simulink model "Lab3_PlantModel"  (R2020a)
settings: Solver=VariableStepAuto  StartTime=0.0  StopTime=2  RelTol=1e-3
libraries: fl_lib x12, ee_lib x10, nesl_utility x3, sdl_lib x2
settings Model: Creator=stevi  LastModifiedBy=Minkyun

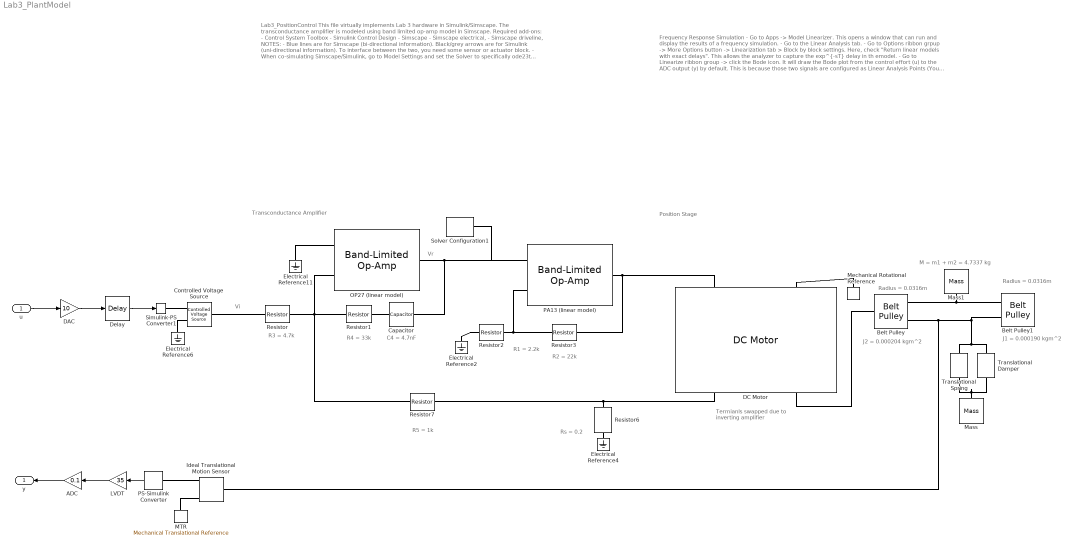
== system Lab3_PlantModel ==
  note: Position Stage
  note: Frequency Response Simulation
      |
      | - Go to Apps -> Model Linearizer. This opens a window that can run and display the results of a frequency simulation.
      | - Go to the Linear Analysis tab.
      | - Go to Options ribbon grpup -> More Options button -> Linearization tab > Block by block settings. Here, check "Return linear models with exact delays". This allows the analyzer to capture the exp^{-sT} delay in th emodel.
      | - Go to Linearize ribbon group -> click the Bode icon.
      |
      | It will draw the Bode plot from the control effort (u) to the ADC output (y) by default. This is because those two signals are configured as Linear Analysis Points (You can see little icons on top of those signal lines). To select input and output locations on block diagram...
      | - Right click on a black/grey simulink signal line. Go to Linear Analysis Points -> Select appropriate types (e.g., open-loop input or open-loop output )
      | - Select different positions for the input and output depending on which frequency response you are interested in.
      | - You just need to select input and output points on the model once and select the analysis you are interested in (e.g., Bode plot, step response, impulse response, nyquist plot, pole-zero plot etc).
      | - Run your analysis, and view the results in this window. By right clicking on the graph, you can add a background grid, change axis limits, change units, and set the phase offset (sometimes the phase will be starting from 360° rather than 0°.
  note: Lab3_PositionControl
      |
      | This file virtually implements Lab 3 hardware in Simulink/Simscape. The transconductance amplifier is modeled using band limited op-amp model in Simscape.
      |
      | Required add-ons:
      | - Control System Toolbox
      | - Simulink Control Design
      | - Simscape
      | - Simscape electrical,
      | - Simscape driveline,
      |
      | NOTES:
      | - Blue lines are for Simscape (bi-directional information). Black/grey arrows are for Simulink (uni-directional information). To interface between the two, you need some sensor or actuator block.
      | - When co-simulating Simscape/Simulink, go to Model Settings and set the Solver to specifically ode23t (mod. stiff/Trapezoidal)
      | - Following recommendation made here: https://www.mathworks.com/help/physmod/simscape/ug/creating-and-simulating-a-simple-model.html
      | - The model simulated fine under the default auto solver selection for an open-loop model, but simulated very slowly for a closed loop model.
  note: Termianls swapped due
      |  to inverting amplifier
  note: Radius = 0.0316m
  note: Vi
  note: J2 = 0.000204 kgm^2
  note: M = m1 + m2 = 4.7337 kg
  note: J1 = 0.000190 kgm^2
  note: Radius = 0.0316m
  note: R5 = 1k
  note: Vr
  note: R4 = 33k
  note: C4 = 4.7nF
  note: R1 = 2.2k
  note: Rs = 0.2
  note: Transconductance Amplifier
  note: R3 = 4.7k
  note: R2 = 22k
  u : Inport
  ADC : Gain  Gain=0.1
  Belt Pulley : sdl_lib/Couplings & Drives/Belt Pulley  belt_type=sdl.enum.belt_type.ideal  sheave_ang=30 deg  num_belts=1  model_f_c=sdl.enum.model_centrifugal.off  linear_density=0.6 kg/m  belt_direction=sdl.enum.belt_direction.opposite  breakable=sdl.enum.max_tension.off  F_max=1e5 N  check_tension=sdl.enum.tension_check.off  r_pulley=0.0316 m  b_pulley=0.01 N*m/(rad/s)  model_inertia=sdl.enum.model_inertia.on  pulley_inertia=0.000204 kg*m^2  initial_velocity=0 rad/s  mu=0.5  phi_wrap=180 deg  v_thr=0.001 m/s
      settings: SourceProductBaseCode=LD  InternalSimscapePortConfiguration="{\"Bottom\":[],\"Left\":[{\"id\":\"S\",\"label\":\"S\",\"type\":\"foundation.mechanical.rotational.rotational\"}],\"Right\":[{\"id\":\"A\",\"label\":\"A\",\"type\":\"foundation.mechanical.translational.translational\"},{\"id\":\"B\",\"label\":\"B\",\"type\":\"foundation.mechanical.translational.translational\"}],\"Top\":[]}"
  Belt Pulley1 : sdl_lib/Couplings & Drives/Belt Pulley  belt_type=sdl.enum.belt_type.ideal  sheave_ang=30 deg  num_belts=1  model_f_c=sdl.enum.model_centrifugal.off  linear_density=0.6 kg/m  belt_direction=sdl.enum.belt_direction.opposite  breakable=sdl.enum.max_tension.off  F_max=1e5 N  check_tension=sdl.enum.tension_check.off  r_pulley=0.0316 m  b_pulley=0.01 N*m/(rad/s)  model_inertia=sdl.enum.model_inertia.on  pulley_inertia=0.000190 kg*m^2  initial_velocity=0 rad/s  mu=0.5  phi_wrap=180 deg  v_thr=0.001 m/s
      settings: SourceProductBaseCode=LD  InternalSimscapePortConfiguration="{\"Bottom\":[],\"Left\":[{\"id\":\"S\",\"label\":\"S\",\"type\":\"foundation.mechanical.rotational.rotational\"}],\"Right\":[{\"id\":\"A\",\"label\":\"A\",\"type\":\"foundation.mechanical.translational.translational\"},{\"id\":\"B\",\"label\":\"B\",\"type\":\"foundation.mechanical.translational.translational\"}],\"Top\":[]}"
  Capacitor : ee_lib/Passive/Capacitor  cap_option=0  c=4.7e-9 F  Cvec=[1e-05, 1e-06] F  Vvec=[0, 10] V  CV_table_symmetry=1  f_vec=[1, 10] kHz  DFext_vec=[.8, 1.2]  C_tol=5  enable_C_tol=0  tol_distribution=1  nSigma=4  r=0 Ohm  g=0 1/Ohm  averaging_period=0 s  enable_operating_limits=0  operating_limit_action=2  max_working_voltage_range=[-25, 25] V  power_rating=1 W  enable_faults=0  fault_action=1  Cscale_faulted=100  R_faulted=1e-3 Ohm  G_faulted=0 1/Ohm  tau_fault=1e-3 s  enable_temporal_fault=0  t_fault=1 s  enable_behavioral_fault=0  max_permissible_voltage_range=[-100, 100] V  t_fail_on_voltage=1 s  i_specify=off  i_priority=None  i=0 A  i_nominal_specify=off  i_nominal_unit=A  i_nominal_value=1  v_specify=off  v_priority=None  v=0 V  v_nominal_specify=off  v_nominal_unit=V  v_nominal_value=1  vc_specify=off  vc_priority=High  vc=0 V  vc_nominal_specify=off  vc_nominal_unit=V  vc_nominal_value=1
  Controlled Voltage Source : fl_lib/Electrical/Electrical Sources/Controlled Voltage Source
  DAC : Gain  Gain=10
  DC Motor : ee_lib/Electromechanical/Brushed Motors/DC Motor  field_option=ee.enum.field_option.pm  Rf=100 Ohm  Lf=1 H  Laf=0.15 H  If0=0 A  parameterization=ee.enum.dcparam_option.circuit_param  Ra=3 Ohm  La=1.07 mH  emf_or_torque=ee.enum.emf_or_torque.ki  Kv=0.072e-3 V/rpm  Ki=0.1963 N*m/A  T_stall=0.24e-3 N*m  w_max=19100 rpm  w_rated=15000 rpm  P_rated=0.08 W  V_rated=1.5 V  J=0.000166 kg*m^2  lam_param=ee.enum.lam_param.damping  lam=0.01 N*m/(rad/s)  i_noload=0 A  V_i_noload=1.5 V  speed0=0 rpm  alpha=3.93e-3 1/K  Tmeas=25 degC  thermal_mass=100 J/K  initial_temperature=25 degC
  Delay : TransportDelay  DelayTime=0.001
  Electrical Reference{2,4,6,11} (4 alike) : fl_lib/Electrical/Electrical Elements/Electrical Reference
  Ideal Translational Motion Sensor : fl_lib/Mechanical/Mechanical Sensors/Ideal Translational Motion Sensor  Tag=Factory Generic  offset=0 m
  LVDT : Gain  Gain=35
  MTR : fl_lib/Mechanical/Translational Elements/Mechanical Translational Reference  Tag=Factory Generic
  Mass : fl_lib/Mechanical/Translational Elements/Mass  mass=4.2882 kg  v_specify=off  v_priority=High  v=0 m/s  v_nominal_specify=off  v_nominal_unit=m/s  v_nominal_value=1  f_specify=off  f_priority=None  f=0 N  f_nominal_specify=off  f_nominal_unit=N  f_nominal_value=1
  Mass1 : fl_lib/Mechanical/Translational Elements/Mass  mass=0.4455 kg  v_specify=off  v_priority=High  v=0 m/s  v_nominal_specify=off  v_nominal_unit=m/s  v_nominal_value=1  f_specify=off  f_priority=None  f=0 N  f_nominal_specify=off  f_nominal_unit=N  f_nominal_value=1
  Mechanical Rotational Reference : fl_lib/Mechanical/Rotational Elements/Mechanical Rotational Reference
  OP27 (linear model) : ee_lib/Integrated Circuits/Band-Limited Op-Amp  A=1778279  Rin=6 MOhm  Rout=70 Ohm  Vmin=-20 V  Vmax=20 V  Vdotmax=2.8*1000*1000 V/s  f=10 Hz  V0=0 V
      settings: SourceProductBaseCode=PS
  PA13 (linear model) : ee_lib/Integrated Circuits/Band-Limited Op-Amp  A=316227  Rin=200 MOhm  Rout=0 Ohm  Vmin=-20 V  Vmax=20 V  Vdotmax=4*1000*1000 V/s  f=100 Hz  V0=0 V
      settings: SourceProductBaseCode=PS
  PS-Simulink Converter : nesl_utility/PS-Simulink Converter  PhysicalDomain=network_engine_domain  SubClassName=ps_output  LeftPortType=input  RightPortType=output  PseudoPeriodic=off  Frequencies=[]  Unit=1  AffineConversion=off
  Resistor : ee_lib/Passive/Resistor  R=4.7*1000 Ohm  R_tol=5  enable_R_tol=0  tol_distribution=1  nSigma=4  enable_operating_limits=0  operating_limit_action=2  max_working_voltage=100 V  power_rating=1 W  enable_faults=0  fault_action=1  R_faulted=inf Ohm  enable_temporal_fault=0  t_fault=1 s  enable_behavioral_fault=0  max_permissible_current=1 A  t_fail_on_current=1 s  noise_mode=0  sample_time=1e-3 s  repeatability=1  auto_seed=1385005866  user_seed=0  Tdevice=25 degC  alpha=3.93e-3 1/K  Tmeas=25 degC  thermal_mass=100 J/K  power_derating_T1=70 degC  power_derating_T2=155 degC  operating_temperature_range_vec=[-50, 150] degC  temperature_specify=off  temperature_priority=High  temperature=298.15 K  temperature_nominal_specify=off  temperature_nominal_unit=K  temperature_nominal_value=1
  Resistor1 : ee_lib/Passive/Resistor  R=33*1000 Ohm  R_tol=5  enable_R_tol=0  tol_distribution=1  nSigma=4  enable_operating_limits=0  operating_limit_action=2  max_working_voltage=100 V  power_rating=1 W  enable_faults=0  fault_action=1  R_faulted=inf Ohm  enable_temporal_fault=0  t_fault=1 s  enable_behavioral_fault=0  max_permissible_current=1 A  t_fail_on_current=1 s  noise_mode=0  sample_time=1e-3 s  repeatability=1  auto_seed=3370429607  user_seed=0  Tdevice=25 degC  alpha=3.93e-3 1/K  Tmeas=25 degC  thermal_mass=100 J/K  power_derating_T1=70 degC  power_derating_T2=155 degC  operating_temperature_range_vec=[-50, 150] degC  temperature_specify=off  temperature_priority=High  temperature=298.15 K  temperature_nominal_specify=off  temperature_nominal_unit=K  temperature_nominal_value=1
  Resistor2 : ee_lib/Passive/Resistor  R=2.2*1000 Ohm  R_tol=5  enable_R_tol=0  tol_distribution=1  nSigma=4  enable_operating_limits=0  operating_limit_action=2  max_working_voltage=100 V  power_rating=1 W  enable_faults=0  fault_action=1  R_faulted=inf Ohm  enable_temporal_fault=0  t_fault=1 s  enable_behavioral_fault=0  max_permissible_current=1 A  t_fail_on_current=1 s  noise_mode=0  sample_time=1e-3 s  repeatability=1  auto_seed=2024463560  user_seed=0  Tdevice=25 degC  alpha=3.93e-3 1/K  Tmeas=25 degC  thermal_mass=100 J/K  power_derating_T1=70 degC  power_derating_T2=155 degC  operating_temperature_range_vec=[-50, 150] degC  temperature_specify=off  temperature_priority=High  temperature=298.15 K  temperature_nominal_specify=off  temperature_nominal_unit=K  temperature_nominal_value=1
  Resistor3 : ee_lib/Passive/Resistor  R=22*1000 Ohm  R_tol=5  enable_R_tol=0  tol_distribution=1  nSigma=4  enable_operating_limits=0  operating_limit_action=2  max_working_voltage=100 V  power_rating=1 W  enable_faults=0  fault_action=1  R_faulted=inf Ohm  enable_temporal_fault=0  t_fault=1 s  enable_behavioral_fault=0  max_permissible_current=1 A  t_fail_on_current=1 s  noise_mode=0  sample_time=1e-3 s  repeatability=1  auto_seed=153599770  user_seed=0  Tdevice=25 degC  alpha=3.93e-3 1/K  Tmeas=25 degC  thermal_mass=100 J/K  power_derating_T1=70 degC  power_derating_T2=155 degC  operating_temperature_range_vec=[-50, 150] degC  temperature_specify=off  temperature_priority=High  temperature=298.15 K  temperature_nominal_specify=off  temperature_nominal_unit=K  temperature_nominal_value=1
  Resistor6 : ee_lib/Passive/Resistor  R=0.2 Ohm  R_tol=5  enable_R_tol=0  tol_distribution=1  nSigma=4  enable_operating_limits=0  operating_limit_action=2  max_working_voltage=100 V  power_rating=1 W  enable_faults=0  fault_action=1  R_faulted=inf Ohm  enable_temporal_fault=0  t_fault=1 s  enable_behavioral_fault=0  max_permissible_current=1 A  t_fail_on_current=1 s  noise_mode=0  sample_time=1e-3 s  repeatability=1  auto_seed=755374864  user_seed=0  Tdevice=25 degC  alpha=3.93e-3 1/K  Tmeas=25 degC  thermal_mass=100 J/K  power_derating_T1=70 degC  power_derating_T2=155 degC  operating_temperature_range_vec=[-50, 150] degC  temperature_specify=off  temperature_priority=High  temperature=298.15 K  temperature_nominal_specify=off  temperature_nominal_unit=K  temperature_nominal_value=1
  Resistor7 : ee_lib/Passive/Resistor  R=1*1000 Ohm  R_tol=5  enable_R_tol=0  tol_distribution=1  nSigma=4  enable_operating_limits=0  operating_limit_action=2  max_working_voltage=100 V  power_rating=1 W  enable_faults=0  fault_action=1  R_faulted=inf Ohm  enable_temporal_fault=0  t_fault=1 s  enable_behavioral_fault=0  max_permissible_current=1 A  t_fail_on_current=1 s  noise_mode=0  sample_time=1e-3 s  repeatability=1  auto_seed=3099927149  user_seed=0  Tdevice=25 degC  alpha=3.93e-3 1/K  Tmeas=25 degC  thermal_mass=100 J/K  power_derating_T1=70 degC  power_derating_T2=155 degC  operating_temperature_range_vec=[-50, 150] degC  temperature_specify=off  temperature_priority=High  temperature=298.15 K  temperature_nominal_specify=off  temperature_nominal_unit=K  temperature_nominal_value=1
  Simulink-PS Converter1 : nesl_utility/Simulink-PS Converter  PhysicalDomain=network_engine_domain  SubClassName=ps_input  LeftPortType=input  RightPortType=output  PseudoPeriodic=off  Frequencies=[]  NoiseDistribution=none  NoiseParameters=[]  Unit=1  AffineConversion=off  FilteringAndDerivatives=provide  SimscapeFilterOrder=1  InputFilterTimeConstant=0.001  UdotUserProvided=0
  Solver Configuration1 : nesl_utility/Solver Configuration  PhysicalDomain=network_engine_domain  SubClassName=solver  LeftPortType=input  RightPortType=generic  Tones=[]  Harmonics=[]  SimulateNoise=off  Profile=off  UseLocalSampling=off  EnableSwitchedLinearOptims=on  FrequencyDomain=off  UseCCode=off  RelTol=0.001  AbsTol=1e-06  MinStep=1e-09  ToWorkspace=off  RevertToSquareIcSolve=off  NumHomotopyIterations=100  PhasorMode=off  PhasorModeNumHarmonics=1  DoDC=on  ResidualTolerance=1e-09  UseLocalSolver=off  LocalSolverChoice=NE_BACKWARD_EULER_ADVANCER  LocalSolverSampleTime=0.00001  DoFixedCost=off  MaxNonlinIter=3  MaxModeIter=2  LinearAlgebra=auto  EquationFormulation=NE_TIME_EF  DelaysMemoryBudget=1024  AutomaticFiltering=off  FilteringTimeConstant=1  PartitionStorageMethod=AS_NEEDED  PartitionMemoryBudget=1024  PartitionMethod=ROBUST
  Translational Damper : fl_lib/Mechanical/Translational Elements/Translational Damper  D=500 N/(m/s)  v_specify=off  v_priority=None  v=0 m/s  v_nominal_specify=off  v_nominal_unit=m/s  v_nominal_value=1  f_specify=off  f_priority=None  f=0 N  f_nominal_specify=off  f_nominal_unit=N  f_nominal_value=1
  Translational Spring : fl_lib/Mechanical/Translational Elements/Translational Spring  spr_rate=500000 N/m  v_specify=off  v_priority=None  v=0 m/s  v_nominal_specify=off  v_nominal_unit=m/s  v_nominal_value=1  f_specify=off  f_priority=None  f=0 N  f_nominal_specify=off  f_nominal_unit=N  f_nominal_value=1  x_specify=off  x_priority=High  x=0 m  x_nominal_specify=off  x_nominal_unit=m  x_nominal_value=1
  y : Outport
  wires:
  u/1 -> DAC/1
  ADC/1 -> y/1
  LVDT/1 -> ADC/1
  DAC/1 -> Delay/1
  Delay/1 -> Simulink-PS Converter1/1
  PS-Simulink Converter/1 -> LVDT/1
  connections:
  Controlled Voltage Source/LConn1 -- Resistor/LConn1
  Mechanical Rotational Reference/LConn1 -- DC Motor/RConn2
  Resistor7/LConn1 -- DC Motor/LConn1 -- Resistor6/LConn1
  Resistor3/RConn1 -- PA13 (linear model)/LConn2 -- Resistor2/LConn1
  OP27 (linear model)/RConn1 -- Solver Configuration1/RConn1 -- PA13 (linear model)/LConn1 -- Capacitor/LConn1
  OP27 (linear model)/LConn2 -- Resistor7/RConn1 -- Resistor1/RConn1 -- Resistor/RConn1
  OP27 (linear model)/LConn1 -- Electrical Reference11/LConn1
  Resistor2/RConn1 -- Electrical Reference2/LConn1
  Electrical Reference4/LConn1 -- Resistor6/RConn1
  Resistor1/LConn1 -- Capacitor/RConn1
  DC Motor/RConn1 -- PA13 (linear model)/RConn1 -- Resistor3/LConn1
  Controlled Voltage Source/RConn2 -- Electrical Reference6/LConn1
  Simulink-PS Converter1/RConn1 -- Controlled Voltage Source/RConn1
  Belt Pulley/LConn1 -- DC Motor/LConn2
  Ideal Translational Motion Sensor/RConn1 -- MTR/LConn1
  Ideal Translational Motion Sensor/RConn3 -- PS-Simulink Converter/LConn1
  Belt Pulley1/RConn1 -- Mass1/LConn1 -- Belt Pulley/RConn1
  Belt Pulley1/RConn2 -- Belt Pulley/RConn2 -- Ideal Translational Motion Sensor/LConn1 -- Translational Damper/LConn1 -- Translational Spring/LConn1
  Translational Spring/RConn1 -- Translational Damper/RConn1 -- Mass/LConn1
